simulink model "final_steady_24a"  (R2025a)
settings: Solver=ode15s  StartTime=0.0  StopTime=14000  RelTol=1e-3
undefined symbols (not defined in the file): bp_er, bp_mf, bp_speed, Cp_rad, epsilon, ETAT_table, m_ratio_bp, PR_table, speed_bp, table_eff, table_mf, theta
(part 2 of 2)

== matlab function final_steady_24a/IHX/IHX_region_1/Lithium_Properties_hot ==
  data: T_h1_average input; P_c input; cp output
function cp = Lithium_Properties_hot(T_h1_average, P_c)
% 热侧液锂比热容。
% 为保持原有两个输入端口和连线不变，保留 P_c；
% 液锂物性使用设计压力 0.234 MPa。

coder.extrinsic('Lithium_property_simulink');

cp = 0;
[cp, ~, ~, ~, ~, ~] = ...
    Lithium_property_simulink(T_h1_average, 0.234e6);
end

== matlab function final_steady_24a/IHX/IHX_region_2/Lithium_Properties_hot ==
  data: T_h1_average input; P_c input; cp output
function cp = Lithium_Properties_hot(T_h1_average, P_c)
% 热侧液锂比热容。
% 为保持原有两个输入端口和连线不变，保留 P_c；
% 液锂物性使用设计压力 0.234 MPa。

coder.extrinsic('Lithium_property_simulink');

cp = 0;
[cp, ~, ~, ~, ~, ~] = ...
    Lithium_property_simulink(T_h1_average, 0.234e6);
end

== matlab function final_steady_24a/TAC/Compressor/HeXe_Properties (point 1) ==
  data: T_in input; P_in input; gamma output
function gamma = HeXe_Properties_hot(T_in, P_in)
coder.extrinsic('HeXe_property_simulink');
gamma=0;
[~, gamma, ~, ~, ~, ~] = HeXe_property_simulink(T_in, P_in);
end

== matlab function final_steady_24a/IHX/IHX_region_2/HeXe_Properties_cold ==
  data: T_c1_average input; cp output; P_in input
function cp = HeXe_Properties_cold(T_c1_average,P_in)

coder.extrinsic('HeXe_property_simulink');

cp = 0;
[cp, ~, ~, ~, ~, ~] = ...
    HeXe_property_simulink(T_c1_average, P_in);
end

== matlab function final_steady_24a/TAC/Compressor/HeXe_Properties(point 1)1 ==
  data: T_in input; P_in input; cp1 output
function cp1 = HeXe_Properties(T_in, P_in)
coder.extrinsic('HeXe_property_simulink');
cp1 = 0; 
[cp1, ~, ~, ~, ~, ~] = HeXe_property_simulink(T_in, P_in);
end

== matlab function final_steady_24a/TAC/Compressor/HeXe_Properties(point 2s) ==
  data: T5s input; P_out input; cp2 output
function cp2 = HeXe_Properties(T5s, P_out)
coder.extrinsic('HeXe_property_simulink');
cp2 = 0; 
[cp2, ~, ~, ~, ~, ~] = HeXe_property_simulink(T5s, P_out);
end

== matlab function final_steady_24a/TAC/Compressor/MATLAB Function ==
  data: T_in input; r input; T5s output; gamma input
function T5s = fcn(T_in, r, gamma)
T5s = T_in * r^((gamma - 1)/gamma);
end

== matlab function final_steady_24a/recuperator/MannRegion_1/HeXe_Properties_cold ==
  data: T_in input; P_in input; cp output
function cp = HeXe_Properties_cold(T_in, P_in)
% 调用外置函数计算 He-Xe 比热容
coder.extrinsic('HeXe_property_simulink');

cp = 0;                                     % 必须先初始化
[cp, ~, ~, ~, ~, ~] = HeXe_property_simulink(T_in, P_in);  % 调用外部文件
end

== matlab function final_steady_24a/recuperator/MannRegion_1/HeXe_Properties_hot ==
  data: T_in input; P_in input; cp output
function cp = HeXe_Properties_hot(T_in, P_in)
% 调用外置函数计算 He-Xe 比热容
coder.extrinsic('HeXe_property_simulink');

cp = 0;                                     % 必须先初始化
[cp, ~, ~, ~, ~, ~] = HeXe_property_simulink(T_in, P_in);  % 调用外部文件
end

== matlab function final_steady_24a/recuperator/MannRegion_2/HeXe_Properties_cold ==
  data: T_in input; P_in input; cp output
function cp = HeXe_Properties_cold(T_in, P_in)
% 调用外置函数计算 He-Xe 比热容
coder.extrinsic('HeXe_property_simulink');

cp = 0;                                     % 必须先初始化
[cp, ~, ~, ~, ~, ~] = HeXe_property_simulink(T_in, P_in);  % 调用外部文件
end

== matlab function final_steady_24a/recuperator/MannRegion_2/HeXe_Properties_hot ==
  data: T_in input; P_in input; cp output
function cp = HeXe_Properties_hot(T_in, P_in)
% 调用外置函数计算 He-Xe 比热容
coder.extrinsic('HeXe_property_simulink');

cp = 0;                                     % 必须先初始化
[cp, ~, ~, ~, ~, ~] = HeXe_property_simulink(T_in, P_in);  % 调用外部文件
end

== matlab function final_steady_24a/TAC/Compressor/MATLAB Function1 ==
  data: T_out output; T_in input; eta_c input; cp1 input; cp2 input; T5s input
function T_out = Fcn(T_in, eta_c, cp1, cp2, T5s)
T_out = T_in + (cp2*(T5s - T_in))/(cp1*eta_c);
end

== matlab function final_steady_24a/precooler/precooler_1/HeXe_Properties_hot ==
  data: T_in input; P_in input; cp output
function cp = HeXe_Properties_hot(T_in, P_in)
% 调用外置函数计算 He-Xe 比热容
coder.extrinsic('HeXe_property_simulink');

cp = 0;                                     % 必须先初始化
[cp, ~, ~, ~, ~, ~] = HeXe_property_simulink(T_in, P_in);  % 调用外部文件
end

== matlab function final_steady_24a/precooler/precooler_1/NaK_Properties_cold ==
  data: T_in input; cp output
function cp = NaK_Properties_cold(T_in)
cp = 1000.*(1.061 - 3.694e-4.*T_in + 4.615e-8.*T_in.^2 + 1.509e-10.*T_in.^3);
end

== matlab function final_steady_24a/precooler/precooler_2/HeXe_Properties_hot ==
  data: T_in input; P_in input; cp output
function cp = HeXe_Properties_hot(T_in, P_in)
% 调用外置函数计算 He-Xe 比热容
coder.extrinsic('HeXe_property_simulink');

cp = 0;                                     % 必须先初始化
[cp, ~, ~, ~, ~, ~] = HeXe_property_simulink(T_in, P_in);  % 调用外部文件
end

== matlab function final_steady_24a/precooler/precooler_2/NaK_Properties_cold1 ==
  data: T_in input; cp output
function cp = NaK_Properties_cold(T_in)
cp = 1000.*(1.061 - 3.694e-4.*T_in + 4.615e-8.*T_in.^2 + 1.509e-10.*T_in.^3);
end

== matlab function final_steady_24a/rediator/MATLAB Function ==
  data: T input; Cp output
function Cp = Cp_h(T)
Cp = 1000.*(1.061 - 3.694e-4.*T + 4.615e-8.*T.^2 + 1.509e-10.*T.^3);
end

== matlab function final_steady_24a/TAC/Turbine/HeXe_Properties (point 1) ==
  data: T_in input; P_in input; gamma output
function gamma = HeXe_Properties_hot(T_in, P_in)
% 调用外置函数计算 He-Xe 比热容
coder.extrinsic('HeXe_property_simulink');
gamma=0;
[~, gamma, ~, ~, ~, ~] = HeXe_property_simulink(T_in, P_in);  % 调用外部文件
end

== matlab function final_steady_24a/TAC/Turbine/HeXe_Properties(point 1) ==
  data: T_in input; P_in input; cp1 output
function cp1 = HeXe_Properties(T_in, P_in)
% 调用外置函数计算 He-Xe 比热容
coder.extrinsic('HeXe_property_simulink');
cp1 = 0; 
[cp1, ~, ~, ~, ~, ~] = HeXe_property_simulink(T_in, P_in);  % 调用外部文件
end

== matlab function final_steady_24a/TAC/Turbine/HeXe_Properties(point 2s) ==
  data: T_in input; P_in input; cp2 output
function cp2 = HeXe_Properties(T_in, P_in)
% 调用外置函数计算 He-Xe 比热容
coder.extrinsic('HeXe_property_simulink');
cp2 = 0; 
[cp2, ~, ~, ~, ~, ~] = HeXe_property_simulink(T_in, P_in);  % 调用外部文件
end

== matlab function final_steady_24a/TAC/Turbine/MATLAB Function ==
  data: pi input; T2s output; phi input; T1 input
function T2s = fcn(pi, phi, T1)
    T2s = T1 * pi^(-phi);
end

== matlab function final_steady_24a/TAC/Turbine/MATLAB Function1 ==
  data: T2 output; T1 input; neta input; cp1 input; cp2 input; T2s input
function T2= Fcn(T1,neta,cp1,cp2,T2s)
T2=T1-(neta*cp2*(T1-T2s))/cp1;
end
